simulink model "ct_reorder_van_core"  (R2013a)
settings: Solver=ode45  StartTime=0.0  StopTime=5000  RelTol=1e-3
libraries: xbsIndex_r4 x320, casper_library_reorder x4, casper_library_delays x1, ox_lib x1
(part 3 of 3)

== system ct_reorder_van_core/one_ant_a_time/square_transposer3/barrel_switcher ==
  sel : Inport
  sync_in : Inport  Port=2
  In1 : Inport  Port=3
  In2 : Inport  Port=4
  Delay_sync : xbsIndex_r4/Delay  rst=off  infoeditControl=Selection of Reset will increase slice count due to use of real FFs and instead of SRLs  en=off  latency=1  dbl_ovrd=off  reg_retiming=on  block_type=delay
  Mux11 : xbsIndex_r4/Mux  inputs=2  en=off  latency=1  precision=Full  arith_type=Unsigned  n_bits=16  bin_pt=14  quantization=Truncate  overflow=Wrap  dbl_ovrd=off  block_type=mux
  Mux21 : xbsIndex_r4/Mux  inputs=2  en=off  latency=1  precision=Full  arith_type=Unsigned  n_bits=16  bin_pt=14  quantization=Truncate  overflow=Wrap  dbl_ovrd=off  block_type=mux
  Slice1 : xbsIndex_r4/Slice  nbits=1  boolean_output=off  mode=Upper Bit Location + Width  bit1=-0  base1=MSB of Input  bit0=0  base0=LSB of Input  dbl_ovrd=off  block_type=slice
  sync_out : Outport
  Out1 : Outport  Port=2
  Out2 : Outport  Port=3
  wires:
  sync_in/1 -> Delay_sync/1
  Delay_sync/1 -> sync_out/1
  sel/1 -> Slice1/1
  Slice1/1 -> Mux11/1, Mux21/1
  In1/1 -> Mux11/2, Mux21/3
  Mux11/1 -> Out1/1
  In2/1 -> Mux21/2, Mux11/3
  Mux21/1 -> Out2/1

== system ct_reorder_van_core/one_ant_a_time/square_transposer3/db0 ==
  din : Inport
  delay : xbsIndex_r4/Delay  rst=off  infoeditControl=Selection of Reset will increase slice count due to use of real FFs and instead of SRLs  en=off  latency=DelayLen  dbl_ovrd=off  reg_retiming=on  block_type=delay
  dout : Outport
  wires:
  din/1 -> delay/1
  delay/1 -> dout/1

== system ct_reorder_van_core/one_ant_a_time/square_transposer3/df1 ==
  din : Inport
  delay : xbsIndex_r4/Delay  rst=off  infoeditControl=Selection of Reset will increase slice count due to use of real FFs and instead of SRLs  en=off  latency=DelayLen  dbl_ovrd=off  reg_retiming=on  block_type=delay
  dout : Outport
  wires:
  din/1 -> delay/1
  delay/1 -> dout/1

== system ct_reorder_van_core/one_ant_a_time/square_transposer3/dsync ==
  din : Inport
  delay : xbsIndex_r4/Delay  rst=off  infoeditControl=Selection of Reset will increase slice count due to use of real FFs and instead of SRLs  en=off  latency=DelayLen  dbl_ovrd=off  reg_retiming=on  block_type=delay
  dout : Outport
  wires:
  din/1 -> delay/1
  delay/1 -> dout/1

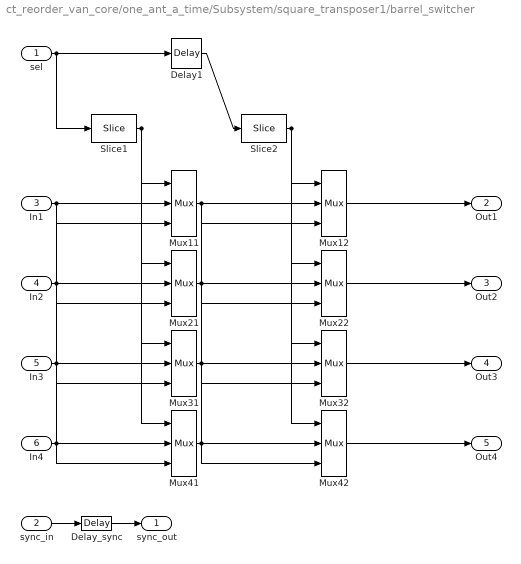
== system ct_reorder_van_core/one_ant_a_time/Subsystem/square_transposer1/barrel_switcher ==
  sel : Inport
  sync_in : Inport  Port=2
  In1 : Inport  Port=3
  In2 : Inport  Port=4
  In3 : Inport  Port=5
  In4 : Inport  Port=6
  Delay1 : xbsIndex_r4/Delay  rst=off  infoeditControl=Selection of Reset will increase slice count due to use of real FFs and instead of SRLs  en=off  latency=1  dbl_ovrd=off  reg_retiming=on  block_type=delay
  Delay_sync : xbsIndex_r4/Delay  rst=off  infoeditControl=Selection of Reset will increase slice count due to use of real FFs and instead of SRLs  en=off  latency=2  dbl_ovrd=off  reg_retiming=on  block_type=delay
  Mux{11..12,21..22,31..32,41..42} (8 alike) : xbsIndex_r4/Mux  inputs=2  en=off  latency=1  precision=Full  arith_type=Unsigned  n_bits=16  bin_pt=14  quantization=Truncate  overflow=Wrap  dbl_ovrd=off  block_type=mux
  Slice1 : xbsIndex_r4/Slice  nbits=1  boolean_output=off  mode=Upper Bit Location + Width  bit1=-0  base1=MSB of Input  bit0=0  base0=LSB of Input  dbl_ovrd=off  block_type=slice
  Slice2 : xbsIndex_r4/Slice  nbits=1  boolean_output=off  mode=Upper Bit Location + Width  bit1=-1  base1=MSB of Input  bit0=0  base0=LSB of Input  dbl_ovrd=off  block_type=slice
  sync_out : Outport
  Out1 : Outport  Port=2
  Out2 : Outport  Port=3
  Out3 : Outport  Port=4
  Out4 : Outport  Port=5
  wires:
  sync_in/1 -> Delay_sync/1
  Delay_sync/1 -> sync_out/1
  sel/1 -> Slice1/1, Delay1/1
  Delay1/1 -> Slice2/1
  Slice1/1 -> Mux11/1, Mux21/1, Mux31/1, Mux41/1
  Slice2/1 -> Mux12/1, Mux22/1, Mux32/1, Mux42/1
  In1/1 -> Mux11/2, Mux31/3
  Mux12/1 -> Out1/1
  In2/1 -> Mux21/2, Mux41/3
  Mux22/1 -> Out2/1
  In3/1 -> Mux31/2, Mux11/3
  Mux32/1 -> Out3/1
  In4/1 -> Mux41/2, Mux21/3
  Mux42/1 -> Out4/1
  Mux11/1 -> Mux12/2, Mux42/3
  Mux21/1 -> Mux22/2, Mux12/3
  Mux31/1 -> Mux32/2, Mux22/3
  Mux41/1 -> Mux42/2, Mux32/3

== system ct_reorder_van_core/one_ant_a_time/Subsystem/square_transposer1/db0 ==
  din : Inport
  delay : xbsIndex_r4/Delay  rst=off  infoeditControl=Selection of Reset will increase slice count due to use of real FFs and instead of SRLs  en=off  latency=DelayLen  dbl_ovrd=off  reg_retiming=on  block_type=delay
  dout : Outport
  wires:
  din/1 -> delay/1
  delay/1 -> dout/1

== system ct_reorder_van_core/one_ant_a_time/Subsystem/square_transposer1/db1 ==
  din : Inport
  delay : xbsIndex_r4/Delay  rst=off  infoeditControl=Selection of Reset will increase slice count due to use of real FFs and instead of SRLs  en=off  latency=DelayLen  dbl_ovrd=off  reg_retiming=on  block_type=delay
  dout : Outport
  wires:
  din/1 -> delay/1
  delay/1 -> dout/1

== system ct_reorder_van_core/one_ant_a_time/Subsystem/square_transposer1/db2 ==
  din : Inport
  delay : xbsIndex_r4/Delay  rst=off  infoeditControl=Selection of Reset will increase slice count due to use of real FFs and instead of SRLs  en=off  latency=DelayLen  dbl_ovrd=off  reg_retiming=on  block_type=delay
  dout : Outport
  wires:
  din/1 -> delay/1
  delay/1 -> dout/1

== system ct_reorder_van_core/one_ant_a_time/Subsystem/square_transposer1/df1 ==
  din : Inport
  delay : xbsIndex_r4/Delay  rst=off  infoeditControl=Selection of Reset will increase slice count due to use of real FFs and instead of SRLs  en=off  latency=DelayLen  dbl_ovrd=off  reg_retiming=on  block_type=delay
  dout : Outport
  wires:
  delay/1 -> dout/1
  din/1 -> delay/1

== system ct_reorder_van_core/one_ant_a_time/Subsystem/square_transposer1/df2 ==
  din : Inport
  delay : xbsIndex_r4/Delay  rst=off  infoeditControl=Selection of Reset will increase slice count due to use of real FFs and instead of SRLs  en=off  latency=DelayLen  dbl_ovrd=off  reg_retiming=on  block_type=delay
  dout : Outport
  wires:
  din/1 -> delay/1
  delay/1 -> dout/1

== system ct_reorder_van_core/one_ant_a_time/Subsystem/square_transposer1/df3 ==
  din : Inport
  delay : xbsIndex_r4/Delay  rst=off  infoeditControl=Selection of Reset will increase slice count due to use of real FFs and instead of SRLs  en=off  latency=DelayLen  dbl_ovrd=off  reg_retiming=on  block_type=delay
  dout : Outport
  wires:
  din/1 -> delay/1
  delay/1 -> dout/1

== system ct_reorder_van_core/one_ant_a_time/Subsystem/square_transposer1/dsync ==
  din : Inport
  delay : xbsIndex_r4/Delay  rst=off  infoeditControl=Selection of Reset will increase slice count due to use of real FFs and instead of SRLs  en=off  latency=DelayLen  dbl_ovrd=off  reg_retiming=on  block_type=delay
  dout : Outport
  wires:
  din/1 -> delay/1
  delay/1 -> dout/1

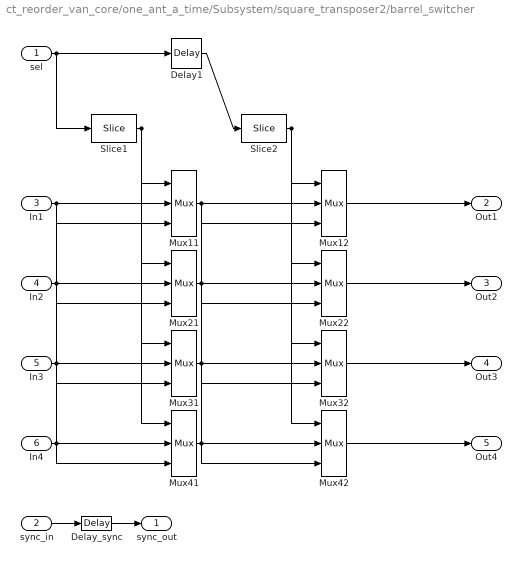
== system ct_reorder_van_core/one_ant_a_time/Subsystem/square_transposer2/barrel_switcher ==
  sel : Inport
  sync_in : Inport  Port=2
  In1 : Inport  Port=3
  In2 : Inport  Port=4
  In3 : Inport  Port=5
  In4 : Inport  Port=6
  Delay1 : xbsIndex_r4/Delay  rst=off  infoeditControl=Selection of Reset will increase slice count due to use of real FFs and instead of SRLs  en=off  latency=1  dbl_ovrd=off  reg_retiming=on  block_type=delay
  Delay_sync : xbsIndex_r4/Delay  rst=off  infoeditControl=Selection of Reset will increase slice count due to use of real FFs and instead of SRLs  en=off  latency=2  dbl_ovrd=off  reg_retiming=on  block_type=delay
  Mux{11..12,21..22,31..32,41..42} (8 alike) : xbsIndex_r4/Mux  inputs=2  en=off  latency=1  precision=Full  arith_type=Unsigned  n_bits=16  bin_pt=14  quantization=Truncate  overflow=Wrap  dbl_ovrd=off  block_type=mux
  Slice1 : xbsIndex_r4/Slice  nbits=1  boolean_output=off  mode=Upper Bit Location + Width  bit1=-0  base1=MSB of Input  bit0=0  base0=LSB of Input  dbl_ovrd=off  block_type=slice
  Slice2 : xbsIndex_r4/Slice  nbits=1  boolean_output=off  mode=Upper Bit Location + Width  bit1=-1  base1=MSB of Input  bit0=0  base0=LSB of Input  dbl_ovrd=off  block_type=slice
  sync_out : Outport
  Out1 : Outport  Port=2
  Out2 : Outport  Port=3
  Out3 : Outport  Port=4
  Out4 : Outport  Port=5
  wires:
  Mux41/1 -> Mux32/3, Mux42/2
  Mux31/1 -> Mux22/3, Mux32/2
  Mux21/1 -> Mux12/3, Mux22/2
  Mux11/1 -> Mux42/3, Mux12/2
  Mux42/1 -> Out4/1
  In4/1 -> Mux21/3, Mux41/2
  Mux32/1 -> Out3/1
  In3/1 -> Mux11/3, Mux31/2
  Mux22/1 -> Out2/1
  In2/1 -> Mux41/3, Mux21/2
  Mux12/1 -> Out1/1
  In1/1 -> Mux31/3, Mux11/2
  Slice2/1 -> Mux42/1, Mux32/1, Mux22/1, Mux12/1
  Slice1/1 -> Mux41/1, Mux31/1, Mux21/1, Mux11/1
  Delay1/1 -> Slice2/1
  sel/1 -> Delay1/1, Slice1/1
  Delay_sync/1 -> sync_out/1
  sync_in/1 -> Delay_sync/1

== system ct_reorder_van_core/one_ant_a_time/Subsystem/square_transposer2/db0 ==
  din : Inport
  delay : xbsIndex_r4/Delay  rst=off  infoeditControl=Selection of Reset will increase slice count due to use of real FFs and instead of SRLs  en=off  latency=DelayLen  dbl_ovrd=off  reg_retiming=on  block_type=delay
  dout : Outport
  wires:
  delay/1 -> dout/1
  din/1 -> delay/1

== system ct_reorder_van_core/one_ant_a_time/Subsystem/square_transposer2/db1 ==
  din : Inport
  delay : xbsIndex_r4/Delay  rst=off  infoeditControl=Selection of Reset will increase slice count due to use of real FFs and instead of SRLs  en=off  latency=DelayLen  dbl_ovrd=off  reg_retiming=on  block_type=delay
  dout : Outport
  wires:
  delay/1 -> dout/1
  din/1 -> delay/1

== system ct_reorder_van_core/one_ant_a_time/Subsystem/square_transposer2/db2 ==
  din : Inport
  delay : xbsIndex_r4/Delay  rst=off  infoeditControl=Selection of Reset will increase slice count due to use of real FFs and instead of SRLs  en=off  latency=DelayLen  dbl_ovrd=off  reg_retiming=on  block_type=delay
  dout : Outport
  wires:
  delay/1 -> dout/1
  din/1 -> delay/1

== system ct_reorder_van_core/one_ant_a_time/Subsystem/square_transposer2/df1 ==
  din : Inport
  delay : xbsIndex_r4/Delay  rst=off  infoeditControl=Selection of Reset will increase slice count due to use of real FFs and instead of SRLs  en=off  latency=DelayLen  dbl_ovrd=off  reg_retiming=on  block_type=delay
  dout : Outport
  wires:
  din/1 -> delay/1
  delay/1 -> dout/1

== system ct_reorder_van_core/one_ant_a_time/Subsystem/square_transposer2/df2 ==
  din : Inport
  delay : xbsIndex_r4/Delay  rst=off  infoeditControl=Selection of Reset will increase slice count due to use of real FFs and instead of SRLs  en=off  latency=DelayLen  dbl_ovrd=off  reg_retiming=on  block_type=delay
  dout : Outport
  wires:
  delay/1 -> dout/1
  din/1 -> delay/1

== system ct_reorder_van_core/one_ant_a_time/Subsystem/square_transposer2/df3 ==
  din : Inport
  delay : xbsIndex_r4/Delay  rst=off  infoeditControl=Selection of Reset will increase slice count due to use of real FFs and instead of SRLs  en=off  latency=DelayLen  dbl_ovrd=off  reg_retiming=on  block_type=delay
  dout : Outport
  wires:
  delay/1 -> dout/1
  din/1 -> delay/1

== system ct_reorder_van_core/one_ant_a_time/Subsystem/square_transposer2/dsync ==
  din : Inport
  delay : xbsIndex_r4/Delay  rst=off  infoeditControl=Selection of Reset will increase slice count due to use of real FFs and instead of SRLs  en=off  latency=DelayLen  dbl_ovrd=off  reg_retiming=on  block_type=delay
  dout : Outport
  wires:
  delay/1 -> dout/1
  din/1 -> delay/1

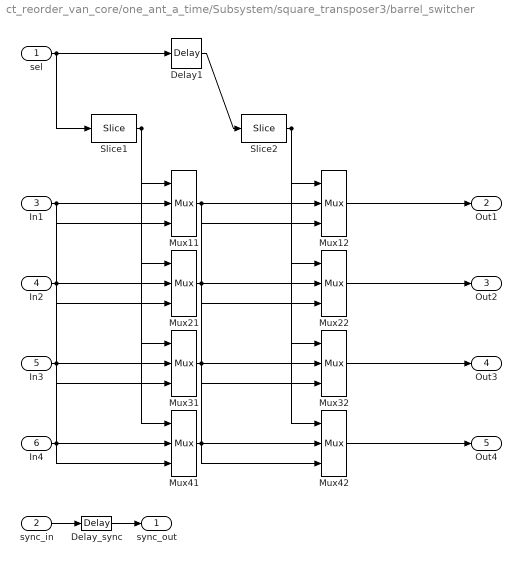
== system ct_reorder_van_core/one_ant_a_time/Subsystem/square_transposer3/barrel_switcher ==
  sel : Inport
  sync_in : Inport  Port=2
  In1 : Inport  Port=3
  In2 : Inport  Port=4
  In3 : Inport  Port=5
  In4 : Inport  Port=6
  Delay1 : xbsIndex_r4/Delay  rst=off  infoeditControl=Selection of Reset will increase slice count due to use of real FFs and instead of SRLs  en=off  latency=1  dbl_ovrd=off  reg_retiming=on  block_type=delay
  Delay_sync : xbsIndex_r4/Delay  rst=off  infoeditControl=Selection of Reset will increase slice count due to use of real FFs and instead of SRLs  en=off  latency=2  dbl_ovrd=off  reg_retiming=on  block_type=delay
  Mux{11..12,21..22,31..32,41..42} (8 alike) : xbsIndex_r4/Mux  inputs=2  en=off  latency=1  precision=Full  arith_type=Unsigned  n_bits=16  bin_pt=14  quantization=Truncate  overflow=Wrap  dbl_ovrd=off  block_type=mux
  Slice1 : xbsIndex_r4/Slice  nbits=1  boolean_output=off  mode=Upper Bit Location + Width  bit1=-0  base1=MSB of Input  bit0=0  base0=LSB of Input  dbl_ovrd=off  block_type=slice
  Slice2 : xbsIndex_r4/Slice  nbits=1  boolean_output=off  mode=Upper Bit Location + Width  bit1=-1  base1=MSB of Input  bit0=0  base0=LSB of Input  dbl_ovrd=off  block_type=slice
  sync_out : Outport
  Out1 : Outport  Port=2
  Out2 : Outport  Port=3
  Out3 : Outport  Port=4
  Out4 : Outport  Port=5
  wires:
  Mux41/1 -> Mux32/3, Mux42/2
  Mux31/1 -> Mux22/3, Mux32/2
  Mux21/1 -> Mux12/3, Mux22/2
  Mux11/1 -> Mux42/3, Mux12/2
  Mux42/1 -> Out4/1
  In4/1 -> Mux21/3, Mux41/2
  Mux32/1 -> Out3/1
  In3/1 -> Mux11/3, Mux31/2
  Mux22/1 -> Out2/1
  In2/1 -> Mux41/3, Mux21/2
  Mux12/1 -> Out1/1
  In1/1 -> Mux31/3, Mux11/2
  Slice2/1 -> Mux42/1, Mux32/1, Mux22/1, Mux12/1
  Slice1/1 -> Mux41/1, Mux31/1, Mux21/1, Mux11/1
  Delay1/1 -> Slice2/1
  sel/1 -> Delay1/1, Slice1/1
  Delay_sync/1 -> sync_out/1
  sync_in/1 -> Delay_sync/1

== system ct_reorder_van_core/one_ant_a_time/Subsystem/square_transposer3/db0 ==
  din : Inport
  delay : xbsIndex_r4/Delay  rst=off  infoeditControl=Selection of Reset will increase slice count due to use of real FFs and instead of SRLs  en=off  latency=DelayLen  dbl_ovrd=off  reg_retiming=on  block_type=delay
  dout : Outport
  wires:
  delay/1 -> dout/1
  din/1 -> delay/1

== system ct_reorder_van_core/one_ant_a_time/Subsystem/square_transposer3/db1 ==
  din : Inport
  delay : xbsIndex_r4/Delay  rst=off  infoeditControl=Selection of Reset will increase slice count due to use of real FFs and instead of SRLs  en=off  latency=DelayLen  dbl_ovrd=off  reg_retiming=on  block_type=delay
  dout : Outport
  wires:
  delay/1 -> dout/1
  din/1 -> delay/1

== system ct_reorder_van_core/one_ant_a_time/Subsystem/square_transposer3/db2 ==
  din : Inport
  delay : xbsIndex_r4/Delay  rst=off  infoeditControl=Selection of Reset will increase slice count due to use of real FFs and instead of SRLs  en=off  latency=DelayLen  dbl_ovrd=off  reg_retiming=on  block_type=delay
  dout : Outport
  wires:
  delay/1 -> dout/1
  din/1 -> delay/1

== system ct_reorder_van_core/one_ant_a_time/Subsystem/square_transposer3/df1 ==
  din : Inport
  delay : xbsIndex_r4/Delay  rst=off  infoeditControl=Selection of Reset will increase slice count due to use of real FFs and instead of SRLs  en=off  latency=DelayLen  dbl_ovrd=off  reg_retiming=on  block_type=delay
  dout : Outport
  wires:
  din/1 -> delay/1
  delay/1 -> dout/1

== system ct_reorder_van_core/one_ant_a_time/Subsystem/square_transposer3/df2 ==
  din : Inport
  delay : xbsIndex_r4/Delay  rst=off  infoeditControl=Selection of Reset will increase slice count due to use of real FFs and instead of SRLs  en=off  latency=DelayLen  dbl_ovrd=off  reg_retiming=on  block_type=delay
  dout : Outport
  wires:
  delay/1 -> dout/1
  din/1 -> delay/1

== system ct_reorder_van_core/one_ant_a_time/Subsystem/square_transposer3/df3 ==
  din : Inport
  delay : xbsIndex_r4/Delay  rst=off  infoeditControl=Selection of Reset will increase slice count due to use of real FFs and instead of SRLs  en=off  latency=DelayLen  dbl_ovrd=off  reg_retiming=on  block_type=delay
  dout : Outport
  wires:
  delay/1 -> dout/1
  din/1 -> delay/1

== system ct_reorder_van_core/one_ant_a_time/Subsystem/square_transposer3/dsync ==
  din : Inport
  delay : xbsIndex_r4/Delay  rst=off  infoeditControl=Selection of Reset will increase slice count due to use of real FFs and instead of SRLs  en=off  latency=DelayLen  dbl_ovrd=off  reg_retiming=on  block_type=delay
  dout : Outport
  wires:
  delay/1 -> dout/1
  din/1 -> delay/1

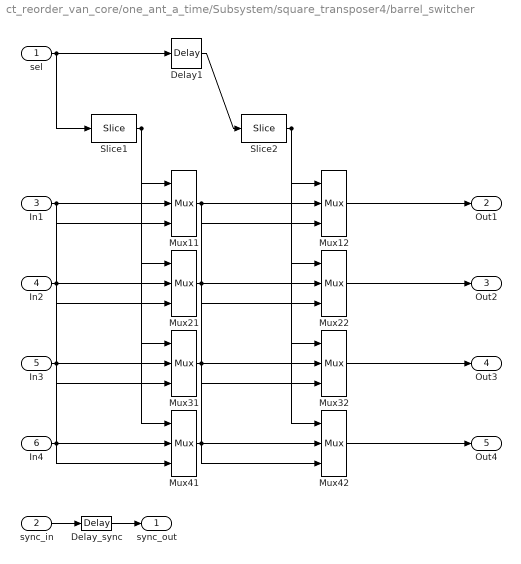
== system ct_reorder_van_core/one_ant_a_time/Subsystem/square_transposer4/barrel_switcher ==
  sel : Inport
  sync_in : Inport  Port=2
  In1 : Inport  Port=3
  In2 : Inport  Port=4
  In3 : Inport  Port=5
  In4 : Inport  Port=6
  Delay1 : xbsIndex_r4/Delay  rst=off  infoeditControl=Selection of Reset will increase slice count due to use of real FFs and instead of SRLs  en=off  latency=1  dbl_ovrd=off  reg_retiming=on  block_type=delay
  Delay_sync : xbsIndex_r4/Delay  rst=off  infoeditControl=Selection of Reset will increase slice count due to use of real FFs and instead of SRLs  en=off  latency=2  dbl_ovrd=off  reg_retiming=on  block_type=delay
  Mux{11..12,21..22,31..32,41..42} (8 alike) : xbsIndex_r4/Mux  inputs=2  en=off  latency=1  precision=Full  arith_type=Unsigned  n_bits=16  bin_pt=14  quantization=Truncate  overflow=Wrap  dbl_ovrd=off  block_type=mux
  Slice1 : xbsIndex_r4/Slice  nbits=1  boolean_output=off  mode=Upper Bit Location + Width  bit1=-0  base1=MSB of Input  bit0=0  base0=LSB of Input  dbl_ovrd=off  block_type=slice
  Slice2 : xbsIndex_r4/Slice  nbits=1  boolean_output=off  mode=Upper Bit Location + Width  bit1=-1  base1=MSB of Input  bit0=0  base0=LSB of Input  dbl_ovrd=off  block_type=slice
  sync_out : Outport
  Out1 : Outport  Port=2
  Out2 : Outport  Port=3
  Out3 : Outport  Port=4
  Out4 : Outport  Port=5
  wires:
  sync_in/1 -> Delay_sync/1
  Delay_sync/1 -> sync_out/1
  sel/1 -> Slice1/1, Delay1/1
  Delay1/1 -> Slice2/1
  Slice1/1 -> Mux11/1, Mux21/1, Mux31/1, Mux41/1
  Slice2/1 -> Mux12/1, Mux22/1, Mux32/1, Mux42/1
  In1/1 -> Mux11/2, Mux31/3
  Mux12/1 -> Out1/1
  In2/1 -> Mux21/2, Mux41/3
  Mux22/1 -> Out2/1
  In3/1 -> Mux31/2, Mux11/3
  Mux32/1 -> Out3/1
  In4/1 -> Mux41/2, Mux21/3
  Mux42/1 -> Out4/1
  Mux11/1 -> Mux12/2, Mux42/3
  Mux21/1 -> Mux22/2, Mux12/3
  Mux31/1 -> Mux32/2, Mux22/3
  Mux41/1 -> Mux42/2, Mux32/3

== system ct_reorder_van_core/one_ant_a_time/Subsystem/square_transposer4/db0 ==
  din : Inport
  delay : xbsIndex_r4/Delay  rst=off  infoeditControl=Selection of Reset will increase slice count due to use of real FFs and instead of SRLs  en=off  latency=DelayLen  dbl_ovrd=off  reg_retiming=on  block_type=delay
  dout : Outport
  wires:
  din/1 -> delay/1
  delay/1 -> dout/1

== system ct_reorder_van_core/one_ant_a_time/Subsystem/square_transposer4/db1 ==
  din : Inport
  delay : xbsIndex_r4/Delay  rst=off  infoeditControl=Selection of Reset will increase slice count due to use of real FFs and instead of SRLs  en=off  latency=DelayLen  dbl_ovrd=off  reg_retiming=on  block_type=delay
  dout : Outport
  wires:
  din/1 -> delay/1
  delay/1 -> dout/1

== system ct_reorder_van_core/one_ant_a_time/Subsystem/square_transposer4/db2 ==
  din : Inport
  delay : xbsIndex_r4/Delay  rst=off  infoeditControl=Selection of Reset will increase slice count due to use of real FFs and instead of SRLs  en=off  latency=DelayLen  dbl_ovrd=off  reg_retiming=on  block_type=delay
  dout : Outport
  wires:
  din/1 -> delay/1
  delay/1 -> dout/1

== system ct_reorder_van_core/one_ant_a_time/Subsystem/square_transposer4/df1 ==
  din : Inport
  delay : xbsIndex_r4/Delay  rst=off  infoeditControl=Selection of Reset will increase slice count due to use of real FFs and instead of SRLs  en=off  latency=DelayLen  dbl_ovrd=off  reg_retiming=on  block_type=delay
  dout : Outport
  wires:
  delay/1 -> dout/1
  din/1 -> delay/1

== system ct_reorder_van_core/one_ant_a_time/Subsystem/square_transposer4/df2 ==
  din : Inport
  delay : xbsIndex_r4/Delay  rst=off  infoeditControl=Selection of Reset will increase slice count due to use of real FFs and instead of SRLs  en=off  latency=DelayLen  dbl_ovrd=off  reg_retiming=on  block_type=delay
  dout : Outport
  wires:
  din/1 -> delay/1
  delay/1 -> dout/1

== system ct_reorder_van_core/one_ant_a_time/Subsystem/square_transposer4/df3 ==
  din : Inport
  delay : xbsIndex_r4/Delay  rst=off  infoeditControl=Selection of Reset will increase slice count due to use of real FFs and instead of SRLs  en=off  latency=DelayLen  dbl_ovrd=off  reg_retiming=on  block_type=delay
  dout : Outport
  wires:
  din/1 -> delay/1
  delay/1 -> dout/1

== system ct_reorder_van_core/one_ant_a_time/Subsystem/square_transposer4/dsync ==
  din : Inport
  delay : xbsIndex_r4/Delay  rst=off  infoeditControl=Selection of Reset will increase slice count due to use of real FFs and instead of SRLs  en=off  latency=DelayLen  dbl_ovrd=off  reg_retiming=on  block_type=delay
  dout : Outport
  wires:
  din/1 -> delay/1
  delay/1 -> dout/1

== system ct_reorder_van_core/one_ant_a_time/reorder0/addr_replicate/bussify ==
  in1 : Inport
  in2 : Inport  Port=2
  in3 : Inport  Port=3
  in4 : Inport  Port=4
  concatenate : xbsIndex_r4/Concat  num_inputs=4  dbl_ovrd=off  block_type=concat
  reinterpret{1..4} (4 alike) : xbsIndex_r4/Reinterpret  force_arith_type=on  arith_type=Unsigned  force_bin_pt=on  bin_pt=0  block_type=reinterpret
      reinterpret1 settings: infoedit="Changes signal type without altering the binary representation.   You can changed the signal between signed and unsigned, and relocate the binary point.<br><br>Hardware notes: In hardware this block costs nothing.<br><br>Example:  Suppose the input is 6 bits wide, signed, with 2 fractional bits, and the output is forced to unsigned with 0 fractional bits.  Then an input of -2.0 (1110.00 in binary 2's complement) becomes an output of 56 (111000 in binary)."
  bus_out : Outport
  wires:
  concatenate/1 -> bus_out/1
  in1/1 -> reinterpret1/1
  reinterpret1/1 -> concatenate/1
  in2/1 -> reinterpret2/1
  reinterpret2/1 -> concatenate/2
  in3/1 -> reinterpret3/1
  reinterpret3/1 -> concatenate/3
  in4/1 -> reinterpret4/1
  reinterpret4/1 -> concatenate/4
